simulink model "control"  (R2021b)
settings: Solver=VariableStepAuto  StartTime=0.0  StopTime=10.0  RelTol=1e-3
settings Model: Creator=Li Chong  LastModifiedBy=Li Chong

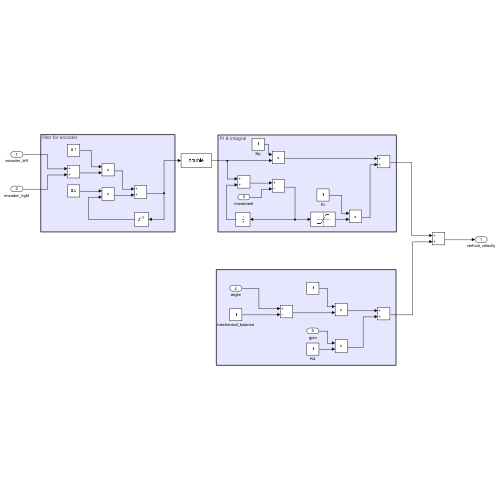
[thumbnail: Simulink's stored preview of the top-level diagram]
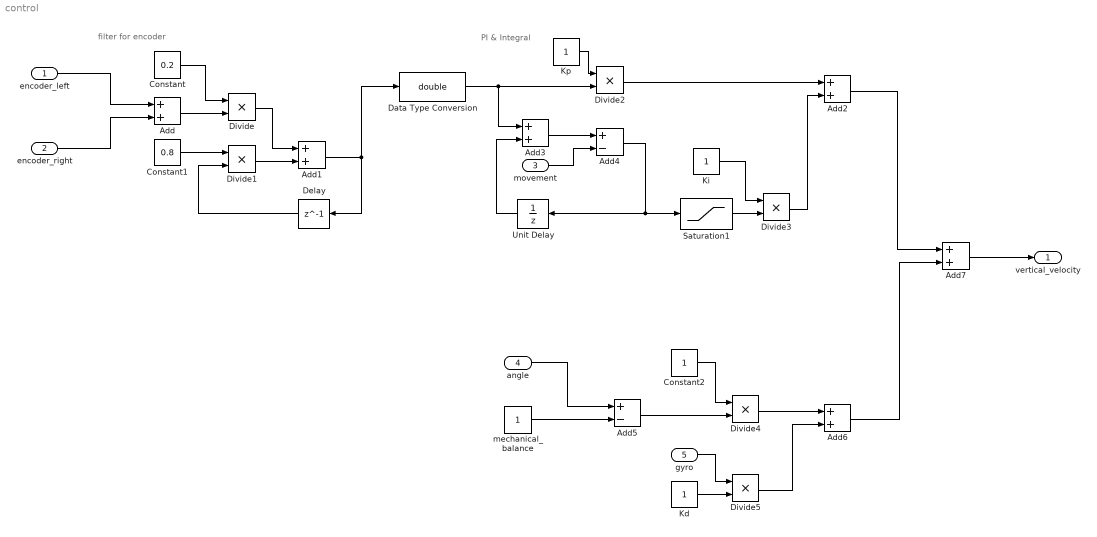
== system control ==
  note: PI & Integral
  note: filter for encoder
  encoder_left : Inport
  encoder_right : Inport  Port=2
  movement : Inport  Port=3
  angle : Inport  Port=4
  gyro : Inport  Port=5
  Add{,1..3,6..7} (6 alike) : Sum
  Add4 : Sum  Inputs=+-
  Add5 : Sum  Inputs=+-
  Constant : Constant  Value=0.2
  Constant1 : Constant  Value=0.8
  Constant2 : Constant
  Data Type Conversion : DataTypeConversion  OutDataTypeStr=double
  Delay : Delay  DelayLength=1  InitialCondition=0
  Divide{,1..5} (6 alike) : Product  Inputs=**
  Kd : Constant
  Ki : Constant
  Kp : Constant
  Saturation1 : Saturate  UpperLimit=10000  LowerLimit=-10000
  Unit Delay : UnitDelay  SampleTime=-1  HasFrameUpgradeWarning=on
  mechanical_balance : Constant
  vertical_velocity : Outport
  wires:
  encoder_left/1 -> Add/1
  encoder_right/1 -> Add/2
  Add/1 -> Divide/2
  Constant/1 -> Divide/1
  Divide/1 -> Add1/1
  Constant1/1 -> Divide1/1
  Add1/1 -> Data Type Conversion/1, Delay/1
  Divide1/1 -> Add1/2
  Delay/1 -> Divide1/2
  Kp/1 -> Divide2/1
  Data Type Conversion/1 -> Add3/1, Divide2/2
  Divide2/1 -> Add2/1
  Add2/1 -> Add7/1
  Unit Delay/1 -> Add3/2
  Saturation1/1 -> Divide3/2
  Divide3/1 -> Add2/2
  Add3/1 -> Add4/1
  movement/1 -> Add4/2
  Add4/1 -> Saturation1/1, Unit Delay/1
  Ki/1 -> Divide3/1
  angle/1 -> Add5/1
  mechanical_balance/1 -> Add5/2
  Add5/1 -> Divide4/2
  Constant2/1 -> Divide4/1
  Divide4/1 -> Add6/1
  gyro/1 -> Divide5/1
  Kd/1 -> Divide5/2
  Divide5/1 -> Add6/2
  Add6/1 -> Add7/2
  Add7/1 -> vertical_velocity/1
